simulink model "Discharge_FinalModel"  (R2023b)
settings: Solver=FixedStepAuto  StartTime=0.0  StopTime=180  FixedStep=0.01  MaxStep=0.2  RelTol=1e-3
model workspace (MAT data in the model file):
  Agg_Material.Water = 3
  Agg_Material.Cement = 2
  Agg_percent_req = 0.6
  Cement_Material.Water = 3
  Cement_Material.Agg = 1
  Cement_percent_req = 0.6
  Con1.state = 0
  Mass_Agg = Simulink.Parameter
  Mass_Agg.Value = 60
  Mass_Agg.DataType = 'auto'
  Mass_Agg.Complexity = 'real'
  Mass_Agg.Dimensions = [1 1]
  Mass_Cement = 45
  Mass_Water = Simulink.Parameter
  Mass_Water.Value = 70
  Mass_Water.DataType = 'auto'
  Mass_Water.Complexity = 'real'
  Mass_Water.Dimensions = [1 1]
  Requested_Agg_Mode.Associated = 3
  Requested_Agg_Mode.Discharge = 2
  Requested_Agg_Mode.Waiting = 1
  Requested_Cement_Mode.Associated = 3
  Requested_Cement_Mode.Discharge = 2
  Requested_Cement_Mode.Waiting = 1
  Requested_Water_Mode.Associated = 3
  Requested_Water_Mode.Discharge = 2
  Requested_Water_Mode.Waiting = 1
  Scenario = Simulink.SimulationData.Dataset
  Scenario.any.Name = ''
  Scenario.any.Version = 3
  Scenario.any.Storage = Simulink.SimulationData.Storage.RamDatasetStorage
  Scenario.any.Storage.any.Version = 2
  Scenario.any.Storage.any.Elements{1} = timeseries
  Scenario.any.Storage.any.Elements{1}.Name = 'Signal 1'
  Scenario.any.Storage.any.Elements{1}.DataInfo = tsdata.datametadata
  Scenario.any.Storage.any.Elements{1}.DataInfo.Interpolation = tsdata.interpolation
  Scenario.any.Storage.any.Elements{1}.DataInfo.Interpolation.Fhandle : function handle (value not decoded)
  Scenario.any.Storage.any.Elements{1}.DataInfo.Interpolation.Name = 'linear'
  Scenario.any.Storage.any.Elements{1}.TimeInfo = tsdata.timemetadata
  Scenario.any.Storage.any.Elements{1}.TimeInfo.Length = 6
  Scenario.any.Storage.any.Elements{1}.TimeInfo.DuplicateTimes = 1
  Scenario.any.Storage.any.Elements{1}.TimeInfo.Time_ = [0; 0.5; 0.5; 2; 2; 10]
  Scenario.any.Storage.any.Elements{1}.TimeInfo.Initialized = 1
  Scenario.any.Storage.any.Elements{1}.QualityInfo = tsdata.qualmetadata
  Scenario.any.Storage.any.Elements{1}.Data_ = [0; 0; 1; 1; 0; 0]
  Water_percent_req = 0.6
  cement = Simulink.Parameter
  cement.DataType = 'auto'
  cement.DocUnits = 's'
  cement.Complexity = 'real'
  cement.Dimensions = [0 0]
  out = Simulink.SimulationOutput
  out.Data.tout = [0; 2; 4; 6]
  out.Data.yout = Simulink.SimulationData.Dataset
  out.Data.yout.any.Name = 'yout'
  out.Data.yout.any.Version = 3
  out.Data.yout.any.Storage = Simulink.SimulationData.Storage.RamDatasetStorage
  out.Data.yout.any.Storage.any.Version = 2
  out.Data.yout.any.Storage.any.Elements{1} = Simulink.SimulationData.Signal
  out.Data.yout.any.Storage.any.Elements{1}.Version = 1
  out.Data.yout.any.Storage.any.Elements{1}.BlockPath = Simulink.SimulationData.BlockPath
  out.Data.yout.any.Storage.any.Elements{1}.BlockPath.path = {'discharge_to_mixer/time_for_emptying_Agg'}
  out.Data.yout.any.Storage.any.Elements{1}.Values = timeseries
  out.Data.yout.any.Storage.any.Elements{1}.Values.DataInfo = tsdata.datametadata
  out.Data.yout.any.Storage.any.Elements{1}.Values.DataInfo.Interpolation = tsdata.interpolation
  out.Data.yout.any.Storage.any.Elements{1}.Values.DataInfo.Interpolation.Fhandle : function handle (value not decoded)
  out.Data.yout.any.Storage.any.Elements{1}.Values.DataInfo.Interpolation.Name = 'zoh'
  out.Data.yout.any.Storage.any.Elements{1}.Values.TimeInfo = tsdata.timemetadata
  out.Data.yout.any.Storage.any.Elements{1}.Values.TimeInfo.Length = 1
  out.Data.yout.any.Storage.any.Elements{1}.Values.TimeInfo.DuplicateTimes = 0
  out.Data.yout.any.Storage.any.Elements{1}.Values.TimeInfo.Time_ = 0
  out.Data.yout.any.Storage.any.Elements{1}.Values.TimeInfo.Initialized = 1
  out.Data.yout.any.Storage.any.Elements{1}.Values.QualityInfo = tsdata.qualmetadata
  out.Data.yout.any.Storage.any.Elements{1}.Values.Data_ = 26.6666666667
  out.Data.yout.any.Storage.any.Elements{2} = Simulink.SimulationData.Signal
  out.Data.yout.any.Storage.any.Elements{2}.Version = 1
  out.Data.yout.any.Storage.any.Elements{2}.BlockPath = Simulink.SimulationData.BlockPath
  out.Data.yout.any.Storage.any.Elements{2}.BlockPath.path = {'discharge_to_mixer/time_for_emptying_water'}
  out.Data.yout.any.Storage.any.Elements{2}.Values = timeseries
  out.Data.yout.any.Storage.any.Elements{2}.Values.DataInfo = tsdata.datametadata
  out.Data.yout.any.Storage.any.Elements{2}.Values.DataInfo.Interpolation = tsdata.interpolation
  out.Data.yout.any.Storage.any.Elements{2}.Values.DataInfo.Interpolation.Fhandle : function handle (value not decoded)
  out.Data.yout.any.Storage.any.Elements{2}.Values.DataInfo.Interpolation.Name = 'zoh'
  out.Data.yout.any.Storage.any.Elements{2}.Values.TimeInfo = tsdata.timemetadata
  out.Data.yout.any.Storage.any.Elements{2}.Values.TimeInfo.Length = 1
  out.Data.yout.any.Storage.any.Elements{2}.Values.TimeInfo.DuplicateTimes = 0
  out.Data.yout.any.Storage.any.Elements{2}.Values.TimeInfo.Time_ = 0
  out.Data.yout.any.Storage.any.Elements{2}.Values.TimeInfo.Initialized = 1
  out.Data.yout.any.Storage.any.Elements{2}.Values.QualityInfo = tsdata.qualmetadata
  out.Data.yout.any.Storage.any.Elements{2}.Values.Data_ = 26.6666666667
  out.Data.yout.any.Storage.any.Elements{3} = Simulink.SimulationData.Signal
  out.Data.yout.any.Storage.any.Elements{3}.Version = 1
  out.Data.yout.any.Storage.any.Elements{3}.BlockPath = Simulink.SimulationData.BlockPath
  out.Data.yout.any.Storage.any.Elements{3}.BlockPath.path = {'discharge_to_mixer/Output'}
  out.Data.yout.any.Storage.any.Elements{3}.Values = timeseries
  out.Data.yout.any.Storage.any.Elements{3}.Values.Name = 'timecement'
  out.Data.yout.any.Storage.any.Elements{3}.Values.DataInfo = tsdata.datametadata
  out.Data.yout.any.Storage.any.Elements{3}.Values.DataInfo.Units = Simulink.SimulationData.Unit
  out.Data.yout.any.Storage.any.Elements{3}.Values.DataInfo.Units.Name = 's'
  out.Data.yout.any.Storage.any.Elements{3}.Values.DataInfo.Interpolation = tsdata.interpolation
  out.Data.yout.any.Storage.any.Elements{3}.Values.DataInfo.Interpolation.Fhandle : function handle (value not decoded)
  out.Data.yout.any.Storage.any.Elements{3}.Values.DataInfo.Interpolation.Name = 'zoh'
  out.Data.yout.any.Storage.any.Elements{3}.Values.TimeInfo = tsdata.timemetadata
  out.Data.yout.any.Storage.any.Elements{3}.Values.TimeInfo.Length = 1
  out.Data.yout.any.Storage.any.Elements{3}.Values.TimeInfo.DuplicateTimes = 0
  out.Data.yout.any.Storage.any.Elements{3}.Values.TimeInfo.Time_ = 0
  out.Data.yout.any.Storage.any.Elements{3}.Values.TimeInfo.Initialized = 1
  out.Data.yout.any.Storage.any.Elements{3}.Values.QualityInfo = tsdata.qualmetadata
  out.Data.yout.any.Storage.any.Elements{3}.Values.Data_ = 26.6666666667
  out.Data.yout.any.Storage.any.Elements{3}.Name = 'timecement'
  out.Data.yout.any.Storage.any.Elements{4} = Simulink.SimulationData.Signal
  out.Data.yout.any.Storage.any.Elements{4}.Version = 1
  out.Data.yout.any.Storage.any.Elements{4}.BlockPath = Simulink.SimulationData.BlockPath
  out.Data.yout.any.Storage.any.Elements{4}.BlockPath.path = {'discharge_to_mixer/Out1'}
  out.Data.yout.any.Storage.any.Elements{4}.Values = timeseries
  out.Data.yout.any.Storage.any.Elements{4}.Values.DataInfo = tsdata.datametadata
  out.Data.yout.any.Storage.any.Elements{4}.Values.DataInfo.Interpolation = tsdata.interpolation
  out.Data.yout.any.Storage.any.Elements{4}.Values.DataInfo.Interpolation.Fhandle : function handle (value not decoded)
  out.Data.yout.any.Storage.any.Elements{4}.Values.DataInfo.Interpolation.Name = 'zoh'
  out.Data.yout.any.Storage.any.Elements{4}.Values.TimeInfo = tsdata.timemetadata
  out.Data.yout.any.Storage.any.Elements{4}.Values.TimeInfo.Length = 4
  out.Data.yout.any.Storage.any.Elements{4}.Values.TimeInfo.DuplicateTimes = 0
  out.Data.yout.any.Storage.any.Elements{4}.Values.TimeInfo.Time_ = [0; 2; 4; 6]
  out.Data.yout.any.Storage.any.Elements{4}.Values.TimeInfo.Initialized = 1
  out.Data.yout.any.Storage.any.Elements{4}.Values.QualityInfo = tsdata.qualmetadata
  out.Data.yout.any.Storage.any.Elements{4}.Values.Data_ = [0; 0; 0; 0]
  out.Metadata = Simulink.SimulationMetadata
  out.Metadata.ModelInfo.ModelName = 'discharge_to_mixer'
  out.Metadata.ModelInfo.ModelVersion = '1.13'
  out.Metadata.ModelInfo.ModelFilePath = 'E:\uni\Grad Project\matlab_models\discharge_to_mixer.slx'
  out.Metadata.ModelInfo.UserID = 'Sama_Lenovo'
  out.Metadata.ModelInfo.MachineName = 'DESKTOP-4P9UUOA'
  out.Metadata.ModelInfo.Platform = 'PCWIN64'
  out.Metadata.ModelInfo.ModelStructuralChecksum = [1562727731; 3816537074; 2262580822; 789484347]
  out.Metadata.ModelInfo.SimulationMode = 'normal'
  out.Metadata.ModelInfo.StartTime = 0
  out.Metadata.ModelInfo.StopTime = 8
  out.Metadata.ModelInfo.SolverInfo.Type = 'Variable-Step'
  out.Metadata.ModelInfo.SolverInfo.Solver = 'VariableStepDiscrete'
  out.Metadata.ModelInfo.SolverInfo.MaxStepSize = 2
  out.Metadata.ModelInfo.SimulinkVersion.Name = 'Simulink'
  out.Metadata.ModelInfo.SimulinkVersion.Version = '23.2'
  out.Metadata.ModelInfo.SimulinkVersion.Release = '(R2023b)'
  out.Metadata.ModelInfo.SimulinkVersion.Date = '01-Aug-2023'
  out.Metadata.ModelInfo.LoggingInfo.LoggingToFile = 'off'
  out.Metadata.TimingInfo.WallClockTimestampStart = '2024-09-03 03:34:53'
  out.Metadata.TimingInfo.WallClockTimestampStop = '2024-09-03 03:35:03'
  out.Metadata.TimingInfo.InitializationElapsedWallTime = 0.9705936
  out.Metadata.TimingInfo.ExecutionElapsedWallTime = 0.2350868
  out.Metadata.TimingInfo.TerminationElapsedWallTime = 1.0305101
  out.Metadata.TimingInfo.TotalElapsedWallTime = 2.2361905
  out.Metadata.TimingInfo.ProfilerData = 'Profiler is not enabled'
  out.Metadata.ExecutionInfo.StopEvent = 'StopCommand'
  out.Metadata.ExecutionInfo.StopEventSource = []
  out.Metadata.ExecutionInfo.StopEventDescription = 'Stop command issued at time 8'
  out.Metadata.ExecutionInfo.ErrorDiagnostic = []
  out.Metadata.ExecutionInfo.WarningDiagnostics(1).Diagnostic = MSLDiagnostic
  out.Metadata.ExecutionInfo.WarningDiagnostics(1).Diagnostic.identifier = 'Stateflow:sflint:TransitionShadowingDiagnostic'
  out.Metadata.ExecutionInfo.WarningDiagnostics(1).Diagnostic.message = 'The unconditional transition <a href="matlab:sfprivate(''sfOpenObjectBySId'',''discharge_to_mixer:1:::69'')">''discharge_to_mixer:1:69''</a> prevents execution of other transitions from the same source.
    | 
    | '
  out.Metadata.ExecutionInfo.WarningDiagnostics(1).Diagnostic.arguments{1} = 'The unconditional transition <a href="matlab:sfprivate(''sfOpenObjectBySId'',''discharge_to_mixer:1:::69'')">''discharge_to_mixer:1:69''</a> prevents execution of other transitions from the same source.
    | 
    | '
  out.Metadata.ExecutionInfo.WarningDiagnostics(1).Diagnostic.stack(1).file = 'C:\Program Files\MATLAB\R2023b\toolbox\simulink\core\general\sldiagviewer.p'
  out.Metadata.ExecutionInfo.WarningDiagnostics(1).Diagnostic.stack(1).name = 'sldiagviewer.reportWarning'
  out.Metadata.ExecutionInfo.WarningDiagnostics(1).Diagnostic.stack(1).line = 0
  out.Metadata.ExecutionInfo.WarningDiagnostics(1).Diagnostic.stack(2).file = 'C:\Program Files\MATLAB\R2023b\toolbox\stateflow\stateflow\private\construct_error.m'
  out.Metadata.ExecutionInfo.WarningDiagnostics(1).Diagnostic.stack(2).name = 'construct_error'
  out.Metadata.ExecutionInfo.WarningDiagnostics(1).Diagnostic.stack(2).line = 130
  out.Metadata.ExecutionInfo.WarningDiagnostics(1).Diagnostic.stack(3).file = 'C:\Program Files\MATLAB\R2023b\toolbox\stateflow\stateflow\sfprivate.m'
  out.Metadata.ExecutionInfo.WarningDiagnostics(1).Diagnostic.stack(3).name = 'sfprivate'
  out.Metadata.ExecutionInfo.WarningDiagnostics(1).Diagnostic.stack(3).line = 13
  out.Metadata.ExecutionInfo.WarningDiagnostics(1).Diagnostic.stack(4).file = 'C:\Program Files\MATLAB\R2023b\toolbox\simulink\ui\studio\config\m\+SLStudio\SimulationForwardInDebuggerCB.p'
  out.Metadata.ExecutionInfo.WarningDiagnostics(1).Diagnostic.stack(4).name = 'SimulationForwardInDebuggerCB'
  out.Metadata.ExecutionInfo.WarningDiagnostics(1).Diagnostic.stack(4).line = 0
  out.Metadata.ExecutionInfo.WarningDiagnostics(1).Diagnostic.stack(5).file = 'C:\Program Files\MATLAB\R2023b\toolbox\simulink\ui\studio\config\m\+SLStudio\ToolBars.p'
  out.Metadata.ExecutionInfo.WarningDiagnostics(1).Diagnostic.stack(5).name = 'ToolBars'
  out.Metadata.ExecutionInfo.WarningDiagnostics(1).Diagnostic.stack(5).line = 0
  out.Metadata.ExecutionInfo.WarningDiagnostics(1).Diagnostic.priority = 2
  out.Metadata.ExecutionInfo.WarningDiagnostics(1).SimulationPhase = 'Initialization'
  out.Metadata.ExecutionInfo.WarningDiagnostics(1).SimulationTime = []
  out.Metadata.ExecutionInfo.WarningDiagnostics(2).Diagnostic = MSLDiagnostic
  out.Metadata.ExecutionInfo.WarningDiagnostics(2).Diagnostic.identifier = 'Stateflow:sflint:TransitionToOrFromParallelStateDiagnostic'
  out.Metadata.ExecutionInfo.WarningDiagnostics(2).Diagnostic.message = 'Transition <a href="matlab:sfprivate(''sfOpenObjectBySId'',''discharge_to_mixer:1:::69'')">''discharge_to_mixer:1:69''</a>: Multiple parallel states are entered or exited simultaneously. For more information, <a href="matlab:sfhelp(''stateflow_parallel_state_with_initial_transition_rule'')">click here</a>
    | 
    | '
  out.Metadata.ExecutionInfo.WarningDiagnostics(2).Diagnostic.arguments{1} = 'Transition <a href="matlab:sfprivate(''sfOpenObjectBySId'',''discharge_to_mixer:1:::69'')">''discharge_to_mixer:1:69''</a>: Multiple parallel states are entered or exited simultaneously. For more information, <a href="matlab:sfhelp(''stateflow_parallel_state_with_initial_transition_rule'')">click here</a>
    | 
    | '
  out.Metadata.ExecutionInfo.WarningDiagnostics(2).Diagnostic.stack(1).file = 'C:\Program Files\MATLAB\R2023b\toolbox\simulink\core\general\sldiagviewer.p'
  out.Metadata.ExecutionInfo.WarningDiagnostics(2).Diagnostic.stack(1).name = 'sldiagviewer.reportWarning'
  out.Metadata.ExecutionInfo.WarningDiagnostics(2).Diagnostic.stack(1).line = 0
  out.Metadata.ExecutionInfo.WarningDiagnostics(2).Diagnostic.stack(2).file = 'C:\Program Files\MATLAB\R2023b\toolbox\stateflow\stateflow\private\construct_error.m'
  out.Metadata.ExecutionInfo.WarningDiagnostics(2).Diagnostic.stack(2).name = 'construct_error'
  out.Metadata.ExecutionInfo.WarningDiagnostics(2).Diagnostic.stack(2).line = 130
  out.Metadata.ExecutionInfo.WarningDiagnostics(2).Diagnostic.stack(3).file = 'C:\Program Files\MATLAB\R2023b\toolbox\stateflow\stateflow\sfprivate.m'
  out.Metadata.ExecutionInfo.WarningDiagnostics(2).Diagnostic.stack(3).name = 'sfprivate'
  out.Metadata.ExecutionInfo.WarningDiagnostics(2).Diagnostic.stack(3).line = 13
  out.Metadata.ExecutionInfo.WarningDiagnostics(2).Diagnostic.stack(4).file = 'C:\Program Files\MATLAB\R2023b\toolbox\simulink\ui\studio\config\m\+SLStudio\SimulationForwardInDebuggerCB.p'
  out.Metadata.ExecutionInfo.WarningDiagnostics(2).Diagnostic.stack(4).name = 'SimulationForwardInDebuggerCB'
  out.Metadata.ExecutionInfo.WarningDiagnostics(2).Diagnostic.stack(4).line = 0
  out.Metadata.ExecutionInfo.WarningDiagnostics(2).Diagnostic.stack(5).file = 'C:\Program Files\MATLAB\R2023b\toolbox\simulink\ui\studio\config\m\+SLStudio\ToolBars.p'
  out.Metadata.ExecutionInfo.WarningDiagnostics(2).Diagnostic.stack(5).name = 'ToolBars'
  out.Metadata.ExecutionInfo.WarningDiagnostics(2).Diagnostic.stack(5).line = 0
  out.Metadata.ExecutionInfo.WarningDiagnostics(2).Diagnostic.priority = 2
  out.Metadata.ExecutionInfo.WarningDiagnostics(2).SimulationPhase = 'Initialization'
  out.Metadata.ExecutionInfo.WarningDiagnostics(2).SimulationTime = []
  out.Metadata.ExecutionInfo.WarningDiagnostics(3).Diagnostic = MSLDiagnostic
  out.Metadata.ExecutionInfo.WarningDiagnostics(3).Diagnostic.identifier = 'Stateflow:sflint:TransitionToOrFromParallelStateDiagnostic'
  out.Metadata.ExecutionInfo.WarningDiagnostics(3).Diagnostic.message = 'Transition <a href="matlab:sfprivate(''sfOpenObjectBySId'',''discharge_to_mixer:1:::76'')">''discharge_to_mixer:1:76''</a>: Multiple parallel states are entered or exited simultaneously. For more information, <a href="matlab:sfhelp(''stateflow_parallel_state_with_initial_transition_rule'')">click here</a>
    | 
    | '
  out.Metadata.ExecutionInfo.WarningDiagnostics(3).Diagnostic.arguments{1} = 'Transition <a href="matlab:sfprivate(''sfOpenObjectBySId'',''discharge_to_mixer:1:::76'')">''discharge_to_mixer:1:76''</a>: Multiple parallel states are entered or exited simultaneously. For more information, <a href="matlab:sfhelp(''stateflow_parallel_state_with_initial_transition_rule'')">click here</a>
    | 
    | '
  out.Metadata.ExecutionInfo.WarningDiagnostics(3).Diagnostic.stack(1).file = 'C:\Program Files\MATLAB\R2023b\toolbox\simulink\core\general\sldiagviewer.p'
  out.Metadata.ExecutionInfo.WarningDiagnostics(3).Diagnostic.stack(1).name = 'sldiagviewer.reportWarning'
  out.Metadata.ExecutionInfo.WarningDiagnostics(3).Diagnostic.stack(1).line = 0
  out.Metadata.ExecutionInfo.WarningDiagnostics(3).Diagnostic.stack(2).file = 'C:\Program Files\MATLAB\R2023b\toolbox\stateflow\stateflow\private\construct_error.m'
  out.Metadata.ExecutionInfo.WarningDiagnostics(3).Diagnostic.stack(2).name = 'construct_error'
  out.Metadata.ExecutionInfo.WarningDiagnostics(3).Diagnostic.stack(2).line = 130
  out.Metadata.ExecutionInfo.WarningDiagnostics(3).Diagnostic.stack(3).file = 'C:\Program Files\MATLAB\R2023b\toolbox\stateflow\stateflow\sfprivate.m'
  out.Metadata.ExecutionInfo.WarningDiagnostics(3).Diagnostic.stack(3).name = 'sfprivate'
  out.Metadata.ExecutionInfo.WarningDiagnostics(3).Diagnostic.stack(3).line = 13
  out.Metadata.ExecutionInfo.WarningDiagnostics(3).Diagnostic.stack(4).file = 'C:\Program Files\MATLAB\R2023b\toolbox\simulink\ui\studio\config\m\+SLStudio\SimulationForwardInDebuggerCB.p'
  out.Metadata.ExecutionInfo.WarningDiagnostics(3).Diagnostic.stack(4).name = 'SimulationForwardInDebuggerCB'
  out.Metadata.ExecutionInfo.WarningDiagnostics(3).Diagnostic.stack(4).line = 0
  out.Metadata.ExecutionInfo.WarningDiagnostics(3).Diagnostic.stack(5).file = 'C:\Program Files\MATLAB\R2023b\toolbox\simulink\ui\studio\config\m\+SLStudio\ToolBars.p'
  out.Metadata.ExecutionInfo.WarningDiagnostics(3).Diagnostic.stack(5).name = 'ToolBars'
  out.Metadata.ExecutionInfo.WarningDiagnostics(3).Diagnostic.stack(5).line = 0
  out.Metadata.ExecutionInfo.WarningDiagnostics(3).Diagnostic.priority = 2
  out.Metadata.ExecutionInfo.WarningDiagnostics(3).SimulationPhase = 'Initialization'
  out.Metadata.ExecutionInfo.WarningDiagnostics(3).SimulationTime = []
  out.Metadata.ExecutionInfo.WarningDiagnostics(4).Diagnostic = MSLDiagnostic
  out.Metadata.ExecutionInfo.WarningDiagnostics(4).Diagnostic.identifier = 'Stateflow:sflint:TransitionToOrFromParallelStateDiagnostic'
  out.Metadata.ExecutionInfo.WarningDiagnostics(4).Diagnostic.message = 'Transition <a href="matlab:sfprivate(''sfOpenObjectBySId'',''discharge_to_mixer:1:::92'')">''discharge_to_mixer:1:92''</a>: Multiple parallel states are entered or exited simultaneously. For more information, <a href="matlab:sfhelp(''stateflow_parallel_state_with_initial_transition_rule'')">click here</a>
    | 
    | '
  out.Metadata.ExecutionInfo.WarningDiagnostics(4).Diagnostic.arguments{1} = 'Transition <a href="matlab:sfprivate(''sfOpenObjectBySId'',''discharge_to_mixer:1:::92'')">''discharge_to_mixer:1:92''</a>: Multiple parallel states are entered or exited simultaneously. For more information, <a href="matlab:sfhelp(''stateflow_parallel_state_with_initial_transition_rule'')">click here</a>
    | 
    | '
  out.Metadata.ExecutionInfo.WarningDiagnostics(4).Diagnostic.stack(1).file = 'C:\Program Files\MATLAB\R2023b\toolbox\simulink\core\general\sldiagviewer.p'
  out.Metadata.ExecutionInfo.WarningDiagnostics(4).Diagnostic.stack(1).name = 'sldiagviewer.reportWarning'
  out.Metadata.ExecutionInfo.WarningDiagnostics(4).Diagnostic.stack(1).line = 0
  out.Metadata.ExecutionInfo.WarningDiagnostics(4).Diagnostic.stack(2).file = 'C:\Program Files\MATLAB\R2023b\toolbox\stateflow\stateflow\private\construct_error.m'
  out.Metadata.ExecutionInfo.WarningDiagnostics(4).Diagnostic.stack(2).name = 'construct_error'
  out.Metadata.ExecutionInfo.WarningDiagnostics(4).Diagnostic.stack(2).line = 130
  out.Metadata.ExecutionInfo.WarningDiagnostics(4).Diagnostic.stack(3).file = 'C:\Program Files\MATLAB\R2023b\toolbox\stateflow\stateflow\sfprivate.m'
  out.Metadata.ExecutionInfo.WarningDiagnostics(4).Diagnostic.stack(3).name = 'sfprivate'
  out.Metadata.ExecutionInfo.WarningDiagnostics(4).Diagnostic.stack(3).line = 13
  out.Metadata.ExecutionInfo.WarningDiagnostics(4).Diagnostic.stack(4).file = 'C:\Program Files\MATLAB\R2023b\toolbox\simulink\ui\studio\config\m\+SLStudio\SimulationForwardInDebuggerCB.p'
  out.Metadata.ExecutionInfo.WarningDiagnostics(4).Diagnostic.stack(4).name = 'SimulationForwardInDebuggerCB'
  out.Metadata.ExecutionInfo.WarningDiagnostics(4).Diagnostic.stack(4).line = 0
  out.Metadata.ExecutionInfo.WarningDiagnostics(4).Diagnostic.stack(5).file = 'C:\Program Files\MATLAB\R2023b\toolbox\simulink\ui\studio\config\m\+SLStudio\ToolBars.p'
  out.Metadata.ExecutionInfo.WarningDiagnostics(4).Diagnostic.stack(5).name = 'ToolBars'
  out.Metadata.ExecutionInfo.WarningDiagnostics(4).Diagnostic.stack(5).line = 0
  out.Metadata.ExecutionInfo.WarningDiagnostics(4).Diagnostic.priority = 2
  out.Metadata.ExecutionInfo.WarningDiagnostics(4).SimulationPhase = 'Initialization'
  out.Metadata.ExecutionInfo.WarningDiagnostics(4).SimulationTime = []
  out.Metadata.ExecutionInfo.WarningDiagnostics(5).Diagnostic = MSLDiagnostic
  out.Metadata.ExecutionInfo.WarningDiagnostics(5).Diagnostic.identifier = 'Stateflow:cdr:UnusedDataOrEvent'
  out.Metadata.ExecutionInfo.WarningDiagnostics(5).Diagnostic.message = '<a href="matlab:sfprivate(''sfOpenObjectBySId'',''discharge_to_mixer:1:::67'')">''Cement_precent_req''</a> is defined, but is not used in the Stateflow chart. <a href= "matlab: internal.stateflow.dialogs.UnusedObjectDeleter.createDeleter(''discharge_to_mixer:1:::67'')">Delete this object</a> or <a href= "matlab: sfprivate(''openConfigParamsSFDiagnostics'',21)">configure the diagnostic</a>.
    | 
    | '
  out.Metadata.ExecutionInfo.WarningDiagnostics(5).Diagnostic.arguments{1} = '<a href="matlab:sfprivate(''sfOpenObjectBySId'',''discharge_to_mixer:1:::67'')">''Cement_precent_req''</a> is defined, but is not used in the Stateflow chart. <a href= "matlab: internal.stateflow.dialogs.UnusedObjectDeleter.createDeleter(''discharge_to_mixer:1:::67'')">Delete this object</a> or <a href= "matlab: sfprivate(''openConfigParamsSFDiagnostics'',21)">configure the diagnostic</a>.
    | 
    | '
  out.Metadata.ExecutionInfo.WarningDiagnostics(5).Diagnostic.stack(1).file = 'C:\Program Files\MATLAB\R2023b\toolbox\simulink\core\general\sldiagviewer.p'
  out.Metadata.ExecutionInfo.WarningDiagnostics(5).Diagnostic.stack(1).name = 'sldiagviewer.reportWarning'
  out.Metadata.ExecutionInfo.WarningDiagnostics(5).Diagnostic.stack(1).line = 0
  out.Metadata.ExecutionInfo.WarningDiagnostics(5).Diagnostic.stack(2).file = 'C:\Program Files\MATLAB\R2023b\toolbox\stateflow\stateflow\private\construct_error.m'
  out.Metadata.ExecutionInfo.WarningDiagnostics(5).Diagnostic.stack(2).name = 'construct_error'
  out.Metadata.ExecutionInfo.WarningDiagnostics(5).Diagnostic.stack(2).line = 130
  out.Metadata.ExecutionInfo.WarningDiagnostics(5).Diagnostic.stack(3).file = 'C:\Program Files\MATLAB\R2023b\toolbox\stateflow\stateflow\sfprivate.m'
  out.Metadata.ExecutionInfo.WarningDiagnostics(5).Diagnostic.stack(3).name = 'sfprivate'
  out.Metadata.ExecutionInfo.WarningDiagnostics(5).Diagnostic.stack(3).line = 13
  out.Metadata.ExecutionInfo.WarningDiagnostics(5).Diagnostic.stack(4).file = 'C:\Program Files\MATLAB\R2023b\toolbox\simulink\ui\studio\config\m\+SLStudio\SimulationForwardInDebuggerCB.p'
  out.Metadata.ExecutionInfo.WarningDiagnostics(5).Diagnostic.stack(4).name = 'SimulationForwardInDebuggerCB'
  out.Metadata.ExecutionInfo.WarningDiagnostics(5).Diagnostic.stack(4).line = 0
  out.Metadata.ExecutionInfo.WarningDiagnostics(5).Diagnostic.stack(5).file = 'C:\Program Files\MATLAB\R2023b\toolbox\simulink\ui\studio\config\m\+SLStudio\ToolBars.p'
  out.Metadata.ExecutionInfo.WarningDiagnostics(5).Diagnostic.stack(5).name = 'ToolBars'
  out.Metadata.ExecutionInfo.WarningDiagnostics(5).Diagnostic.stack(5).line = 0
  out.Metadata.ExecutionInfo.WarningDiagnostics(5).Diagnostic.priority = 2
  out.Metadata.ExecutionInfo.WarningDiagnostics(5).SimulationPhase = 'Initialization'
  out.Metadata.ExecutionInfo.WarningDiagnostics(5).SimulationTime = []
  out.Metadata.ExecutionInfo.WarningDiagnostics(6).Diagnostic = MSLDiagnostic
  out.Metadata.ExecutionInfo.WarningDiagnostics(6).Diagnostic.identifier = 'Stateflow:cdr:UnusedDataOrEvent'
  out.Metadata.ExecutionInfo.WarningDiagnostics(6).Diagnostic.message = '<a href="matlab:sfprivate(''sfOpenObjectBySId'',''discharge_to_mixer:1:::63'')">''Cement_percent''</a> is defined, but is not used in the Stateflow chart. <a href= "matlab: internal.stateflow.dialogs.UnusedObjectDeleter.createDeleter(''discharge_to_mixer:1:::63'')">Delete this object</a> or <a href= "matlab: sfprivate(''openConfigParamsSFDiagnostics'',21)">configure the diagnostic</a>.
    | 
    | '
  out.Metadata.ExecutionInfo.WarningDiagnostics(6).Diagnostic.arguments{1} = '<a href="matlab:sfprivate(''sfOpenObjectBySId'',''discharge_to_mixer:1:::63'')">''Cement_percent''</a> is defined, but is not used in the Stateflow chart. <a href= "matlab: internal.stateflow.dialogs.UnusedObjectDeleter.createDeleter(''discharge_to_mixer:1:::63'')">Delete this object</a> or <a href= "matlab: sfprivate(''openConfigParamsSFDiagnostics'',21)">configure the diagnostic</a>.
    | 
    | '
  out.Metadata.ExecutionInfo.WarningDiagnostics(6).Diagnostic.stack(1).file = 'C:\Program Files\MATLAB\R2023b\toolbox\simulink\core\general\sldiagviewer.p'
  out.Metadata.ExecutionInfo.WarningDiagnostics(6).Diagnostic.stack(1).name = 'sldiagviewer.reportWarning'
  out.Metadata.ExecutionInfo.WarningDiagnostics(6).Diagnostic.stack(1).line = 0
  out.Metadata.ExecutionInfo.WarningDiagnostics(6).Diagnostic.stack(2).file = 'C:\Program Files\MATLAB\R2023b\toolbox\stateflow\stateflow\private\construct_error.m'
  out.Metadata.ExecutionInfo.WarningDiagnostics(6).Diagnostic.stack(2).name = 'construct_error'
  out.Metadata.ExecutionInfo.WarningDiagnostics(6).Diagnostic.stack(2).line = 130
  out.Metadata.ExecutionInfo.WarningDiagnostics(6).Diagnostic.stack(3).file = 'C:\Program Files\MATLAB\R2023b\toolbox\stateflow\stateflow\sfprivate.m'
  out.Metadata.ExecutionInfo.WarningDiagnostics(6).Diagnostic.stack(3).name = 'sfprivate'
  out.Metadata.ExecutionInfo.WarningDiagnostics(6).Diagnostic.stack(3).line = 13
  out.Metadata.ExecutionInfo.WarningDiagnostics(6).Diagnostic.stack(4).file = 'C:\Program Files\MATLAB\R2023b\toolbox\simulink\ui\studio\config\m\+SLStudio\SimulationForwardInDebuggerCB.p'
  out.Metadata.ExecutionInfo.WarningDiagnostics(6).Diagnostic.stack(4).name = 'SimulationForwardInDebuggerCB'
  out.Metadata.ExecutionInfo.WarningDiagnostics(6).Diagnostic.stack(4).line = 0
  out.Metadata.ExecutionInfo.WarningDiagnostics(6).Diagnostic.stack(5).file = 'C:\Program Files\MATLAB\R2023b\toolbox\simulink\ui\studio\config\m\+SLStudio\ToolBars.p'
  out.Metadata.ExecutionInfo.WarningDiagnostics(6).Diagnostic.stack(5).name = 'ToolBars'
  out.Metadata.ExecutionInfo.WarningDiagnostics(6).Diagnostic.stack(5).line = 0
  out.Metadata.ExecutionInfo.WarningDiagnostics(6).Diagnostic.priority = 2
  out.Metadata.ExecutionInfo.WarningDiagnostics(6).SimulationPhase = 'Initialization'
  out.Metadata.ExecutionInfo.WarningDiagnostics(6).SimulationTime = []
  out.Metadata.AppInfo = struct()
  rndX = [2; 3]
  state.ON = 1
  state.OFF = 0
  timecement = Simulink.Parameter
  timecement.DataType = 'auto'
  timecement.DocUnits = 's'
  timecement.Complexity = 'real'
  timecement.Dimensions = [0 0]
  water_Material.Agg = 1
  water_Material.Cement = 2
values from neighbouring files (symbols this model uses):
  Agg_Material =     [parameters2.mat]
  Cement_Material =     [parameters2.mat]
  Requested_Agg_Mode =     [parameters2.mat]
  Requested_Cement_Mode =     [parameters2.mat]
  Requested_Water_Mode =     [parameters2.mat]
  water_Material =     [parameters2.mat]
settings Model: PacingRate=2  Creator=Sama_Lenovo  LastModifiedBy=Sama_Lenovo
settings DebuggingCC: BusObjectLabelMismatch=error
settings ConfigComp: PLC_TargetIDE=tiaportal  PLC_GenerateTestbenchDiagCode=on  PLC_MultiTBSigbuilderTimeRange=on  PLC_FoldFBCallOutputVar=off  PLC_RemoveUnusedSSMethodCallArguments=off  PLC_UseCallOutputArgSyntax=off  PLC_EnableUnsignedAndDoubleTypes=off  PLC_EnableUDTSplitting=off  PLC_MaxFieldsInUDT=500  PLC_InlineEnumCastFunction=off

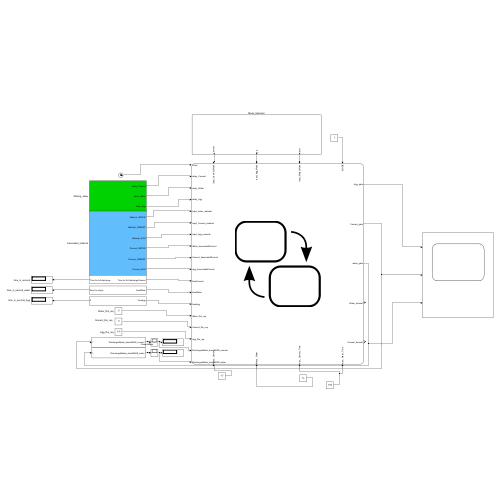
[thumbnail: Simulink's stored preview of the top-level diagram]
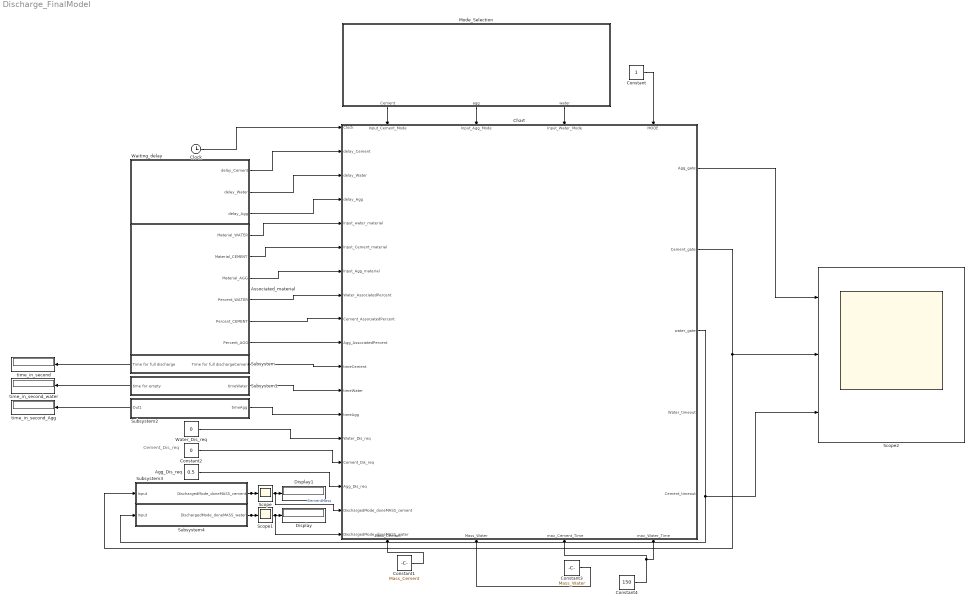
== system Discharge_FinalModel ==
  note: Cement_Dis_req
  Agg_Dis_req : Constant  Value=0.5
  Associated_material : Subsystem  RequirementInfo={} %GIDa_ea989900_2953_4736_9b15_e91975f1d71c
  Chart : Stateflow chart  TreatAsAtomicUnit=on
      settings: PortSchema="{\"entries\":[{\"content\":{\"sides\":[{\"content\":{\"connectorIds\":[\"In2\",\"In13\",\"In14\",\"In12\",\"In10\",\"In8\",\"In6\",\"In11\",\"In1\",\"In25\",\"In16\",\"In17\",\"In15\",\"In19\",\"In20\",\"In21\",\"In3\",\"In4\"]},\"type\":\"ConnectorPlacement.EquallySpacedRectSide\",\"uuid\":\"5f846a4d-3592-4813-aa30-55bca40765f6\"},{\"content\":{\"connectorIds\":[\"Out1\",\"Out2\",\"Out3\",\"Out4\",\"Out5\"],\"side\":\"RIGHT\"},\"type\":\"ConnectorPlacement.EquallySpacedRectSide\",\"uuid\":\"90f2503d-9917-4bdd-921c-fb670f9d6ee2\"},{\"content\":{\"connectorIds\":[\"In7\",\"In5\",\"In9\",\"In18\"],\"side\":\"TOP\"},\"type\":\"ConnectorPlacement.EquallySpacedRectSide\",\"uuid\":\"5e594e37-50f1-4cb8-9f34-9d710cf76db4\"},{\"content\":{\"connectorIds\":[\"In22\",\"In23\",\"In24\",\"In26\"],\"side\":\"BOTTOM\"},\"type\":\"ConnectorPlacement.EquallySpacedRectSide\",\"uuid\":\"4bdbd2b7-6e32-4cc8-ba71-132b52f66466\"}]},\"type\":\"ConnectorPlacement.EquallySpacedConnector\",\"uuid\":\"2322f0f6-1b61-4083-97e0-1fa44badf64c\"}],\"packageUris\":[\"http://schema.mathworks.com/mf0/Connector/R2020b\"],\"version\":\"1.0\"}"
  Clock : Clock
  Constant : Constant
  Constant1 : Constant  Value=Mass_Cement
  Constant2 : Constant  Value=0
  Constant3 : Constant  Value=Mass_Water
  Constant4 : Constant  Value=150
  Display : Display
  Display1 : Display
      settings: RequirementInfo={} %GIDa_52f2f9b7_4820_4635_9f19_044c267ad194
  Mode_Selection : Subsystem  RequirementInfo={} %GIDa_0b8c387b_7712_479f_b037_11126471d815
  Scope : Scope
      settings: RequirementInfo={} %GIDa_ae1336b8_d342_416f_b89e_00177b48e107
  Scope1 : Scope
  Scope2 : Scope  NumInputPorts=3
  Subsystem : Subsystem
      settings: PortSchema="{\"entries\":[{\"content\":{\"sides\":[{\"content\":{\"connectorIds\":[\"Out2\"]},\"type\":\"ConnectorPlacement.EquallySpacedRectSide\",\"uuid\":\"674f9e5e-efc7-4957-abcd-df2b1b1a8339\"},{\"content\":{\"connectorIds\":[\"Out1\"],\"side\":\"RIGHT\"},\"type\":\"ConnectorPlacement.EquallySpacedRectSide\",\"uuid\":\"79a0af93-8dc9-4e0a-bd0b-8564a5d9bfb1\"},{\"content\":{\"side\":\"TOP\"},\"type\":\"ConnectorPlacement.EquallySpacedRectSide\",\"uuid\":\"b1229906-b5e1-49f1-ac96-693991645c64\"}]},\"type\":\"ConnectorPlacement.EquallySpacedConnector\",\"uuid\":\"41521bba-d81f-40aa-a1a2-c88789bee06b\"}],\"packageUris\":[\"http://schema.mathworks.com/mf0/Connector/R2020b\"],\"version\":\"1.0\"}"
  Subsystem1 : Subsystem
      settings: PortSchema="{\"entries\":[{\"content\":{\"sides\":[{\"content\":{\"connectorIds\":[\"Out2\"]},\"type\":\"ConnectorPlacement.EquallySpacedRectSide\",\"uuid\":\"9a186855-5eb2-4958-a818-b3e7ed82ab1d\"},{\"content\":{\"connectorIds\":[\"Out1\"],\"side\":\"RIGHT\"},\"type\":\"ConnectorPlacement.EquallySpacedRectSide\",\"uuid\":\"3a3cf98d-4412-4eec-88b9-49ee45af2032\"},{\"content\":{\"side\":\"TOP\"},\"type\":\"ConnectorPlacement.EquallySpacedRectSide\",\"uuid\":\"6f6469d9-7fcc-47a9-8ccc-5d56ad245aee\"}]},\"type\":\"ConnectorPlacement.EquallySpacedConnector\",\"uuid\":\"654c91bb-487b-4aa4-9a82-d074f04bdc80\"}],\"packageUris\":[\"http://schema.mathworks.com/mf0/Connector/R2020b\"],\"version\":\"1.0\"}"
  Subsystem2 : Subsystem
      settings: PortSchema="{\"entries\":[{\"content\":{\"sides\":[{\"content\":{\"connectorIds\":[\"Out2\"]},\"type\":\"ConnectorPlacement.EquallySpacedRectSide\",\"uuid\":\"9a186855-5eb2-4958-a818-b3e7ed82ab1d\"},{\"content\":{\"connectorIds\":[\"Out1\"],\"side\":\"RIGHT\"},\"type\":\"ConnectorPlacement.EquallySpacedRectSide\",\"uuid\":\"3a3cf98d-4412-4eec-88b9-49ee45af2032\"},{\"content\":{\"side\":\"TOP\"},\"type\":\"ConnectorPlacement.EquallySpacedRectSide\",\"uuid\":\"6f6469d9-7fcc-47a9-8ccc-5d56ad245aee\"}]},\"type\":\"ConnectorPlacement.EquallySpacedConnector\",\"uuid\":\"654c91bb-487b-4aa4-9a82-d074f04bdc80\"}],\"packageUris\":[\"http://schema.mathworks.com/mf0/Connector/R2020b\"],\"version\":\"1.0\"}"
  Subsystem3 : Subsystem
  Subsystem4 : Subsystem
  Waiting_delay : Subsystem  RequirementInfo={} %GIDa_51ce960d_939b_4071_ada2_003032cb31df
  Water_Dis_req : Constant  Value=0
  time_in_second : Display
      settings: RequirementInfo={} %GIDa_3642becf_450a_42d2_9b52_9c521c3eba8b
  time_in_second_Agg : Display
      settings: RequirementInfo={} %GIDa_368e0406_7b4d_4fc7_9f13_e4b09d937ad1
  time_in_second_water : Display
      settings: RequirementInfo={} %GIDa_d99cde4f_e23a_4f57_895f_af2ef083b2f0
  wires:
  Mode_Selection/3(water) -> Chart/9(Input_Water_Mode)
  Mode_Selection/2(agg) -> Chart/5(Input_Agg_Mode)
  Mode_Selection/1(Cement) -> Chart/7(Input_Cement_Mode)
  Clock/1 -> Chart/2(Clock)
  Waiting_delay/1(delay_Cement) -> Chart/13(delay_Cement)
  Waiting_delay/2(delay_Water) -> Chart/14(delay_Water)
  Waiting_delay/3(delay_Agg) -> Chart/12(delay_Agg)
  Associated_material/1(Material_WATER) -> Chart/10(Input_water_material)
  Associated_material/2(Material_CEMENT) -> Chart/8(Input_Cement_material)
  Associated_material/3(Material_AGG) -> Chart/6(Input_Agg_material)
  Associated_material/4(Percent_WATER) -> Chart/11(Water_AssociatedPercent)
  Associated_material/5(Percent_CEMENT) -> Chart/1(Cement_AssociatedPercent)
  Associated_material/6(Percent_AGG) -> Chart/25(Agg_AssociatedPercent)
  Constant/1 -> Chart/18(MODE)
  Subsystem/2(Time for full discharge) -> time_in_second/1
  Subsystem/1(Time for full dischargeCement) -> Chart/16(timeCement)
  Subsystem1/2(time for empty) -> time_in_second_water/1
  Subsystem1/1(timeWater) -> Chart/17(timeWater)
  Subsystem2/2(Out1) -> time_in_second_Agg/1
  Subsystem2/1(timeAgg) -> Chart/15(timeAgg)
  Water_Dis_req/1 -> Chart/19(Water_Dis_req)
  Constant2/1 -> Chart/20(Cement_Dis_req)
  Agg_Dis_req/1 -> Chart/21(Agg_Dis_req)
  Subsystem3/1(DischargedMode_doneMASS_cement) -> Scope/1, Display1/1, Chart/3(DischargedMode_doneMASS_cement)  "CementMass"
  Subsystem4/1(DischargedMode_doneMASS_water) -> Display/1, Chart/4(DischargedMode_doneMASS_water), Scope1/1
  Chart/1(Agg_gate) -> Scope2/1
  Chart/2(Cement_gate) -> Subsystem3/1(Input), Scope2/2
  Chart/3(water_gate) -> Subsystem4/1(Input), Scope2/3
  Constant1/1 -> Chart/22(Mass_Cement)
  Constant3/1 -> Chart/23(Mass_Water)
  Constant4/1 -> Chart/26(max_Water_Time), Chart/24(max_Cement_Time)

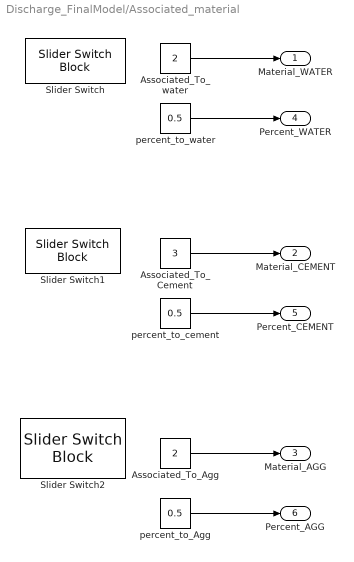
== system Discharge_FinalModel/Associated_material ==
  Associated_To_Agg : Constant  RequirementInfo={} %GIDa_26e499c5_00ff_4f7b_aea6_b4d8bd999c7e  Value=2
  Associated_To_Cement : Constant  RequirementInfo={} %GIDa_54ba17f7_bfdb_4505_9c3d_5c4a3a43e526  Value=3
  Associated_To_water : Constant  RequirementInfo={} %GIDa_68121bd3_5224_46d6_aee8_35862e7ba611  Value=2
  Slider Switch : SliderSwitchBlock  RequirementInfo={} %GIDa_f5f89405_98dd_4e0d_8ff0_dcc3b6252926
      settings: Values={{'Agg', 'Cement'}, [1 2]}
  Slider Switch1 : SliderSwitchBlock  RequirementInfo={} %GIDa_a2737b7f_a805_430e_90b6_18fdfe2f172c
      settings: Values={{'Agg', 'Water'}, [1 3]}
  Slider Switch2 : SliderSwitchBlock  RequirementInfo={} %GIDa_5cec020d_8d62_46c8_8e32_b9133cd81c3e
      settings: Values={{'Water', 'Cement'}, [3 2]}
  percent_to_Agg : Constant  RequirementInfo={} %GIDa_c9a83ccb_b56e_4a03_866b_94f1f2ce3523  Value=0.5
  percent_to_cement : Constant  RequirementInfo={} %GIDa_8f772792_f3a1_4a10_bc21_06f48f3401d4  Value=0.5
  percent_to_water : Constant  RequirementInfo={} %GIDa_0d6611ed_c7b8_4dd4_961c_586f6037ad71  Value=0.5
  Material_WATER : Outport  RequirementInfo={} %GIDa_c1273c22_5413_41ca_9a5b_0cfe3bdf758c
  Material_CEMENT : Outport  RequirementInfo={} %GIDa_bb69f85b_ab28_4d24_b1fb_9cb760ad0f8b  Port=2
  Material_AGG : Outport  RequirementInfo={} %GIDa_6dd6a08e_4aa8_4e22_8a6d_53845be86144  Port=3
  Percent_WATER : Outport  RequirementInfo={} %GIDa_910332db_905b_4c39_88c4_74cc5be45d74  Port=4
  Percent_CEMENT : Outport  RequirementInfo={} %GIDa_82df716c_f9d8_4f07_9368_9773ab747268  Port=5
  Percent_AGG : Outport  RequirementInfo={} %GIDa_4de2a85f_36b1_40c0_aa91_ca24e2e8b23c  Port=6
  wires:
  Associated_To_water/1 -> Material_WATER/1
  Associated_To_Cement/1 -> Material_CEMENT/1
  Associated_To_Agg/1 -> Material_AGG/1
  percent_to_water/1 -> Percent_WATER/1
  percent_to_cement/1 -> Percent_CEMENT/1
  percent_to_Agg/1 -> Percent_AGG/1

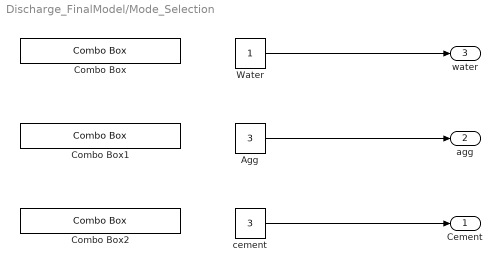
== system Discharge_FinalModel/Mode_Selection ==
  Agg : Constant  RequirementInfo={} %GIDa_286350d6_e5fb_4d7c_a360_635541077f0e  Value=3
  Combo Box : ComboBox  LabelPosition=Hide  SelectedLabel=Waiting
      settings: Values={{'Waiting', 'Discharge', 'Associated'}, [1 2 3]}
  Combo Box1 : ComboBox  LabelPosition=Hide  SelectedLabel=Associated
      settings: Values={{'Waiting', 'Discharge', 'Associated'}, [1 2 3]}
  Combo Box2 : ComboBox  LabelPosition=Hide  SelectedLabel=Associated
      settings: Values={{'Waiting', 'Discharge', 'Associated'}, [1 2 3]}
  Water : Constant  RequirementInfo={} %GIDa_faf9ccc3_cfa9_4946_9fcd_9cc790fb7bed
  cement : Constant  RequirementInfo={} %GIDa_172789b0_11ae_4201_9d0b_478411590e99  Value=3
  Cement : Outport  RequirementInfo={} %GIDa_daccf285_7fea_4113_9e8f_c6cd5b1d0a0c
  agg : Outport  RequirementInfo={} %GIDa_c7bf3833_2d5d_4bda_8d06_3b61f6a221cd  Port=2
  water : Outport  RequirementInfo={} %GIDa_509ac32a_b4b8_4117_a2fd_989faf55c7fd  Port=3
  wires:
  cement/1 -> Cement/1
  Water/1 -> water/1
  Agg/1 -> agg/1

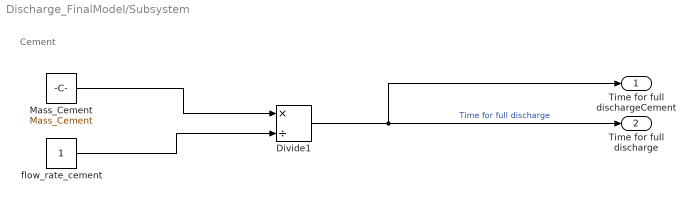
== system Discharge_FinalModel/Subsystem ==
  note: Cement
  Divide1 : Product  RequirementInfo={} %GIDa_533059b9_a879_4113_a61b_3b1b4f3bb3fb  Inputs=*/
  Mass_Cement : Constant  RequirementInfo={} %GIDa_165f97d3_af30_4a9b_8d73_07ffb3e2bd46  Value=Mass_Cement
  flow_rate_cement : Constant  RequirementInfo={} %GIDa_7c48bcf1_dc43_476e_bca7_e7106b08001a
  Time for full dischargeCement : Outport
  Time for full discharge : Outport  Port=2
  wires:
  Divide1/1 -> Time for full discharge/1, Time for full dischargeCement/1  "Time for full discharge"
  flow_rate_cement/1 -> Divide1/2
  Mass_Cement/1 -> Divide1/1

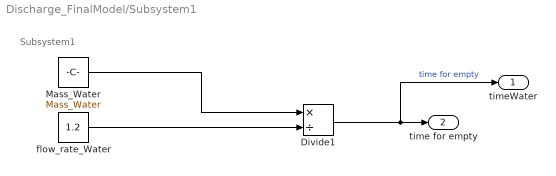
== system Discharge_FinalModel/Subsystem1 ==
  note: Subsystem1
  Divide1 : Product  RequirementInfo={} %GIDa_6e532d37_1212_4999_b26c_4672840bf44a  Inputs=*/
  Mass_Water : Constant  RequirementInfo={} %GIDa_0465f616_9dc8_46b0_868a_0ba91f5c58da  Value=Mass_Water
  flow_rate_Water : Constant  RequirementInfo={} %GIDa_f6ad07e9_4082_44eb_b4f5_c4649e6cfdc5  Value=1.2
  timeWater : Outport
  time for empty : Outport  Port=2
  wires:
  flow_rate_Water/1 -> Divide1/2
  Mass_Water/1 -> Divide1/1
  Divide1/1 -> timeWater/1, time for empty/1  "time for empty"

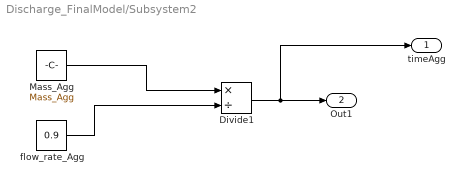
== system Discharge_FinalModel/Subsystem2 ==
  Divide1 : Product  RequirementInfo={} %GIDa_a112a99b_5622_4220_ac20_a4e59fa02c9c  Inputs=*/
  Mass_Agg : Constant  RequirementInfo={} %GIDa_4fd7ddf0_501c_4fef_800b_b2f6b5220781  Value=Mass_Agg
  flow_rate_Agg : Constant  RequirementInfo={} %GIDa_424b0a11_9e48_47f9_aa9b_ac0fe93a4b0a  Value=0.9
  timeAgg : Outport
  Out1 : Outport  Port=2
  wires:
  Mass_Agg/1 -> Divide1/1
  flow_rate_Agg/1 -> Divide1/2
  Divide1/1 -> timeAgg/1, Out1/1

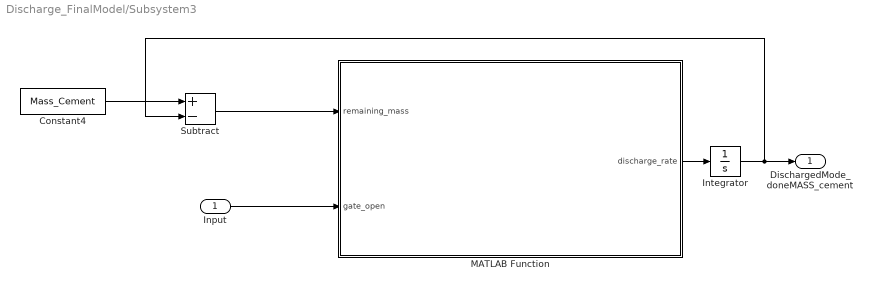
== system Discharge_FinalModel/Subsystem3 ==
  Input : Inport
  Constant4 : Constant  Value=Mass_Cement
  Integrator : Integrator  RequirementInfo={} %GIDa_a735ddd6_9f7d_4141_b286_7267498acf44
  MATLAB Function : MATLAB Function  RequirementInfo={} %GIDa_af0cf62d_8117_4168_ad0f_b8a0836b3db6  TreatAsAtomicUnit=on
  Subtract : Sum  RequirementInfo={} %GIDa_9d245276_18b8_4f36_81c3_849fbe8c1ee1  Inputs=+-
  DischargedMode_doneMASS_cement : Outport
  wires:
  Input/1 -> MATLAB Function/2(gate_open)
  Integrator/1 -> DischargedMode_doneMASS_cement/1, Subtract/2
  MATLAB Function/1(discharge_rate) -> Integrator/1
  Constant4/1 -> Subtract/1
  Subtract/1 -> MATLAB Function/1(remaining_mass)

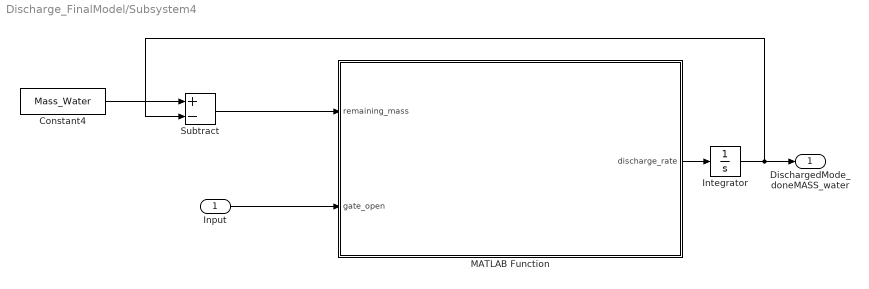
== system Discharge_FinalModel/Subsystem4 ==
  Input : Inport
  Constant4 : Constant  Value=Mass_Water
  Integrator : Integrator
  MATLAB Function : MATLAB Function  TreatAsAtomicUnit=on
  Subtract : Sum  Inputs=+-
  DischargedMode_doneMASS_water : Outport
  wires:
  Input/1 -> MATLAB Function/2(gate_open)
  Integrator/1 -> DischargedMode_doneMASS_water/1, Subtract/2
  MATLAB Function/1(discharge_rate) -> Integrator/1
  Constant4/1 -> Subtract/1
  Subtract/1 -> MATLAB Function/1(remaining_mass)

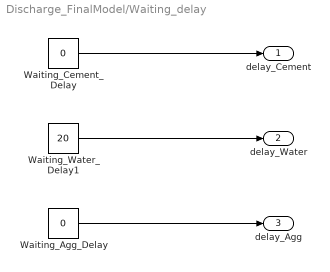
== system Discharge_FinalModel/Waiting_delay ==
  Waiting_Agg_Delay : Constant  RequirementInfo={} %GIDa_59bf980c_6811_4587_a25d_1e1bc46a666c  Value=0
  Waiting_Cement_Delay : Constant  RequirementInfo={} %GIDa_86bf4889_59f8_424e_bdda_339f7ed13cb3  Value=0
  Waiting_Water_Delay1 : Constant  RequirementInfo={} %GIDa_206f2acb_bf51_48ef_b0f5_6958be016af4  Value=20
  delay_Cement : Outport  RequirementInfo={} %GIDa_8d842faf_a196_4b97_8ba3_9205a942752b
  delay_Water : Outport  RequirementInfo={} %GIDa_7a93dbea_9e39_4ab1_bb9c_e485af726ecf  Port=2
  delay_Agg : Outport  RequirementInfo={} %GIDa_d6b30550_1f3f_4a0f_82c1_f3b0a7899949  Port=3
  wires:
  Waiting_Agg_Delay/1 -> delay_Agg/1
  Waiting_Water_Delay1/1 -> delay_Water/1
  Waiting_Cement_Delay/1 -> delay_Cement/1

== stateflow chart Discharge_FinalModel/Chart ==
  state MODE_OF_DISCHARGING [parallel]
    settings: executionOrder=1
    state Time_Based
    state Mass_Based
    (default) -> Time_Based
    Mass_Based -> Time_Based : [MODE == 1]
    Time_Based -> Mass_Based : [MODE == 0]
  state Water1 [parallel]
    settings: executionOrder=2
    state Agg
    state WaterDis
      water_gate = 1;
      Water=1;
      en: WaterON = Clock;
    state Cement
    state water
      en: water_gate = 0;
    state Discharge%
      water_gate = 1;
      en: WaterON = Clock;
      Water=1;
    state CloseGate
      water_gate = 0 ;
    state OpenGate
      water_gate = 1 ;
      Water=1;
      en: WaterON = Clock;
    Water1.Agg -> WaterDis : [(Water_AssociatedPercent*timeAgg)<=Clock-AggON && Agg==1]
    (junction 90) -> Water1.Agg [order 1] : [Input_water_material == water_Material.Agg]
    WaterDis -> Water1.CloseGate [order 2] : [DischargedMode_doneMASS_water >= Mass_Water && in(MODE_OF_DISCHARGING.Mass_Based)]
    WaterDis -> Water1.CloseGate [order 1] : [after(timeWater,sec) && in(MODE_OF_DISCHARGING.Time_Based)]
    Water1.Cement -> WaterDis [order 1] : [(Water_AssociatedPercent*Mass_Cement)<=DischargedMode_doneMASS_cement && Cement == 1&& in(MODE_OF_DISCHARGING.Mass_Based)]
    Water1.Cement -> WaterDis [order 2] : [(Water_AssociatedPercent*timeCement)<=Clock-CementON &&Cement == 1 && in(MODE_OF_DISCHARGING.Time_Based)]
    Water1.Cement -> WaterDis [order 3] : [after(max_Cement_Time*Water_AssociatedPercent,sec) && Cement == 1 && in(MODE_OF_DISCHARGING.Mass_Based) ]{Cement_timeout = 1}
    water -> (junction 90) [order 1] : [Input_Water_Mode == Requested_Water_Mode.Associated]
    (junction 90) -> Water1.Cement [order 2] : [Input_water_material == water_Material.Cement]
    (default) -> water
    water -> Water1.Discharge% [order 2] : [Input_Water_Mode == Requested_Water_Mode.Discharge]
    water -> (junction 92) [order 3] : [Input_Water_Mode == Requested_Water_Mode.Waiting]
    Water1.Discharge% -> Water1.CloseGate [order 3] : [after(max_Water_Time,sec) && in(MODE_OF_DISCHARGING.Mass_Based)]{Water_timeout = 1}
    Water1.Discharge% -> Water1.CloseGate [order 2] : [Water_Dis_req*timeWater<=Clock-WaterON && in(MODE_OF_DISCHARGING.Time_Based)]
    Water1.Discharge% -> Water1.CloseGate [order 1] : [DischargedMode_doneMASS_water >= Mass_Water*Water_Dis_req && in(MODE_OF_DISCHARGING.Mass_Based)]
    Water1.OpenGate -> Water1.CloseGate [order 1] : [after(timeWater,sec) && in(MODE_OF_DISCHARGING.Time_Based)]
    Water1.OpenGate -> Water1.CloseGate [order 2] : [DischargedMode_doneMASS_water >= Mass_Water && in(MODE_OF_DISCHARGING.Mass_Based)]
    Water1.OpenGate -> Water1.CloseGate [order 3] : [after(max_Water_Time,sec) && in(MODE_OF_DISCHARGING.Mass_Based)]{Water_timeout = 1}
    (junction 92) -> Water1.OpenGate : [[after(delay_Water,sec)]]
  state cem [parallel]
    settings: executionOrder=3
    state Agg
    state CementDis
      Cement_gate = 1;
      Cement = 1 ;
      en : CementON = Clock;
    state Water
    state cement
      en: Cement_gate = 0;
    state Discharge%
      Cement_gate = 1;
      Cement=1;
      en : CementON = Clock;
    state OpenGate
      Cement_gate = 1;
      Cement = 1;
      en : CementON = Clock;
    state CloseGate
      Cement_gate = 0;
    cem.Agg -> CementDis : [(Cement_AssociatedPercent*timeAgg)<=Clock-AggON && Agg == 1]
    (junction 121) -> cem.Agg [order 1] : [Input_Cement_material == Cement_Material.Agg]
    CementDis -> cem.CloseGate [order 2] : [DischargedMode_doneMASS_cement >= Mass_Cement && in(MODE_OF_DISCHARGING.Mass_Based)]
    CementDis -> cem.CloseGate [order 1] : [after(timeCement,sec) && in(MODE_OF_DISCHARGING.Time_Based)]
    cem.Water -> CementDis [order 2] : [(Cement_AssociatedPercent*Mass_Water)<=DischargedMode_doneMASS_water && Water == 1 && in(MODE_OF_DISCHARGING.Mass_Based)]
    cem.Water -> CementDis [order 3] : [after(max_Water_Time*Cement_AssociatedPercent,sec) && Cement == 1 && in(MODE_OF_DISCHARGING.Mass_Based) ]{Water_timeout = 1}
    cem.Water -> CementDis [order 1] : [(Cement_AssociatedPercent*timeWater)<=Clock-WaterON && Water == 1 && in(MODE_OF_DISCHARGING.Time_Based)]
    (junction 121) -> cem.Water [order 2] : [Input_Cement_material == Cement_Material.Water]
    cement -> (junction 121) [order 1] : [Input_Cement_Mode == Requested_Cement_Mode.Associated]
    (default) -> cement
    cement -> cem.Discharge% [order 2] : [Input_Cement_Mode == Requested_Cement_Mode.Discharge]
    cement -> (junction 120) [order 3] : [Input_Cement_Mode == Requested_Cement_Mode.Waiting]
    cem.Discharge% -> cem.CloseGate [order 3] : [after(max_Cement_Time,sec) && in(MODE_OF_DISCHARGING.Mass_Based)]{Cement_timeout = 1}
    cem.Discharge% -> cem.CloseGate [order 1] : [Cement_Dis_req <= Clock - CementON  && in(MODE_OF_DISCHARGING.Time_Based)]
    (junction 120) -> cem.OpenGate : [after(delay_Cement,sec)]
    cem.Discharge% -> cem.CloseGate [order 2] : [DischargedMode_doneMASS_cement >= Mass_Cement*Cement_Dis_req && in(MODE_OF_DISCHARGING.Mass_Based)]
    cem.OpenGate -> cem.CloseGate [order 3] : [after(max_Cement_Time,sec) && in(MODE_OF_DISCHARGING.Mass_Based)]{Cement_timeout = 1}
    cem.OpenGate -> cem.CloseGate [order 1] : [after(timeCement,sec) && in(MODE_OF_DISCHARGING.Time_Based)]
    cem.OpenGate -> cem.CloseGate [order 2] : [DischargedMode_doneMASS_cement >= Mass_Cement && in(MODE_OF_DISCHARGING.Mass_Based)]
  state agg [parallel]
    settings: executionOrder=4
    state Cement
    state AggDis
      Agg_gate = 1 ;
      Agg = 1 ;
      en:  AggON = Clock;
    state Water
    state Agg1
      en: Agg_gate = 0;
    state Discharge%
      Agg_gate = 1;
      Agg = 1 ;
      en:  AggON = Clock;
    state OpenGate
      Agg_gate = 1;
      Agg = 1 ;
      en:  AggON = Clock;
    state CloseGate
      Agg_gate = 0;
    agg.Cement -> AggDis [order 1] : [(Agg_AssociatedPercent*timeCement)<=Clock-CementON && Cement == 1 && in(MODE_OF_DISCHARGING.Time_Based) ]
    agg.Cement -> AggDis [order 2] : [(Agg_AssociatedPercent*Mass_Cement)<=DischargedMode_doneMASS_cement && Cement == 1 && in(MODE_OF_DISCHARGING.Mass_Based) ]
    (junction 108) -> agg.Cement [order 1] : [Input_Agg_material == Agg_Material.Cement]
    agg.Cement -> AggDis [order 3] : [after(max_Cement_Time*Agg_AssociatedPercent,sec) && Cement == 1 && in(MODE_OF_DISCHARGING.Mass_Based) ]{Cement_timeout = 1}
    agg.Water -> AggDis [order 1] : [(Agg_AssociatedPercent*timeWater)<=Clock-WaterON && Water == 1]
    agg.Water -> AggDis [order 2] : [(Agg_AssociatedPercent*Mass_Water)<=DischargedMode_doneMASS_water && Water == 1 && in(MODE_OF_DISCHARGING.Mass_Based) ]
    agg.Water -> AggDis [order 3] : [after(max_Water_Time*Agg_AssociatedPercent,sec) && Cement == 1 && in(MODE_OF_DISCHARGING.Mass_Based) ]{Water_timeout = 1}
    AggDis -> agg.CloseGate : [after(timeAgg,sec)]
    Agg1 -> (junction 108) [order 1] : [Input_Agg_Mode == Requested_Agg_Mode.Associated]
    (junction 108) -> agg.Water [order 2] : [Input_Agg_material == Agg_Material.Water]
    Agg1 -> agg.Discharge% [order 2] : [Input_Agg_Mode == Requested_Agg_Mode.Discharge]
    (default) -> Agg1
    Agg1 -> (junction 115) [order 3] : [Input_Agg_Mode == Requested_Agg_Mode.Waiting]
    (junction 115) -> agg.OpenGate : [after(delay_Agg,sec)]
    agg.Discharge% -> agg.CloseGate : [Agg_Dis_req*timeAgg <= Clock - AggON]
    agg.OpenGate -> agg.CloseGate : after(timeAgg,sec)
  data: Cement_AssociatedPercent input; Clock input; DischargedMode_doneMASS_cement input; DischargedMode_doneMASS_water input; Input_Agg_Mode input; Input_Agg_material input; Input_Cement_Mode input; Input_Cement_material input; Input_Water_Mode input; Input_water_material input; Water_AssociatedPercent input; delay_Agg input; delay_Cement input; delay_Water input; timeAgg input; timeCement input; timeWater input; Agg_gate output; Cement_gate output; water_gate output; Agg local =0; AggON local =0; Cement local =0; CementON local =0; Water local =0; WaterON local =0; MODE input; Requested_Water_Mode parameter; water_Material parameter; Requested_Agg_Mode parameter; Requested_Cement_Mode parameter; Agg_Material parameter; Cement_Material parameter; Water_Dis_req input; Cement_Dis_req input; Agg_Dis_req input; Mass_Cement input; Mass_Water input; max_Cement_Time input; Agg_AssociatedPercent input; max_Water_Time input; Water_timeout output; Cement_timeout output

== matlab function Discharge_FinalModel/Subsystem3/MATLAB Function ==
  data: remaining_mass input; discharge_rate output; gate_open input
function discharge_rate = nonLinearDischarge(remaining_mass, gate_open)
    % Ensure remaining_mass is non-negative
    remaining_mass = max(remaining_mass, 0);  % Clamp remaining_mass to zero

    if gate_open == 1 && remaining_mass > 0
        k = 0.75;  % Discharge coefficient, adjust as necessary
        discharge_rate = k * sqrt(remaining_mass);  % Non-linear discharge rate
    else
        discharge_rate = 0;  % No discharge if gate is closed or mass is zero
    end
end

== matlab function Discharge_FinalModel/Subsystem4/MATLAB Function ==
  data: remaining_mass input; discharge_rate output; gate_open input
function discharge_rate = nonLinearDischarge(remaining_mass, gate_open)
    % Ensure remaining_mass is non-negative
    remaining_mass = max(remaining_mass, 0);  % Clamp remaining_mass to zero

    if gate_open == 1 && remaining_mass > 0
        k = 0.5;  % Discharge coefficient, adjust as necessary
        discharge_rate = k * sqrt(remaining_mass);  % Non-linear discharge rate
    else
        discharge_rate = 0;  % No discharge if gate is closed or mass is zero
    end
end
